simulink model "ClosedLoopSystem_PID_Exp_python_block_2"  (R2025b)
settings: Solver=ode1  StartTime=0.0  StopTime=100  FixedStep=Ts  RelTol=1e-3  EnableMultiTasking=on
libraries: simulink_extras x4, sldrtlib x1
(part 2 of 2)

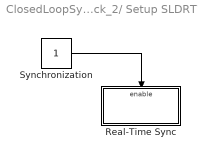
== system ClosedLoopSystem_PID_Exp_python_block_2/ Setup SLDRT1 ==
  Real-Time Sync : Subsystem
  Synchronization : Constant
  wires:
  Synchronization/1 -> Real-Time Sync/Enable

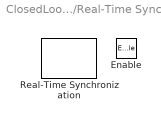
== system ClosedLoopSystem_PID_Exp_python_block_2/ Setup SLDRT1/Real-Time Sync ==
  Enable : EnablePort
  Real-Time Synchronization : sldrtlib/Real-Time Synchronization  SampleTime=Ts  MaxMissedTicks=inf  ShowMissedTicks=off  YieldWhenWaiting=off
